simulink model "RV400_Main_Model"  (R2025b)
settings: Solver=VariableStepAuto  StartTime=0.0  StopTime=100  RelTol=1e-3
libraries: fuzblock x1
settings Model: Creator=lenovo  LastModifiedBy=lenovo

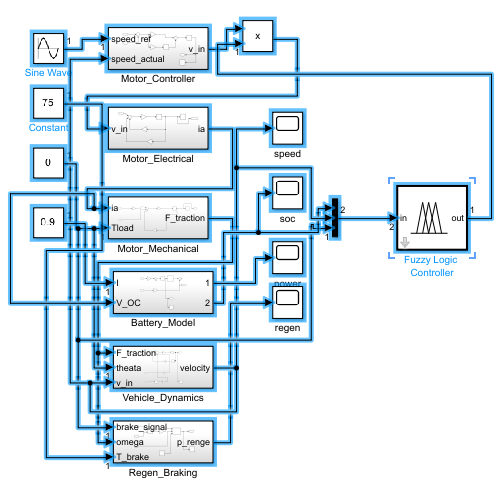
[thumbnail: Simulink's stored preview of the top-level diagram]
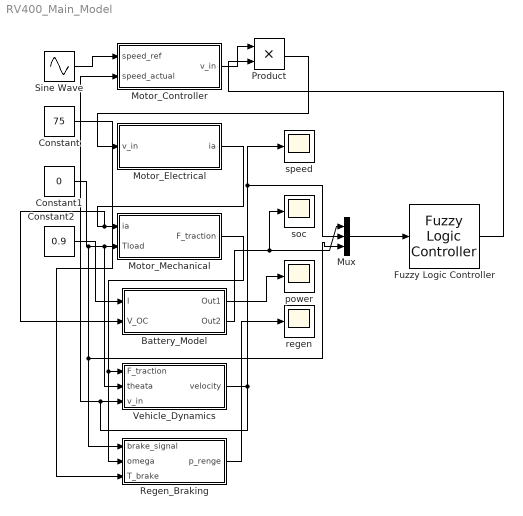
== system RV400_Main_Model ==
  Battery_Model : Subsystem
  Constant : Constant  Value=75
  Constant1 : Constant  Value=0
  Constant2 : Constant  Value=0.9
  Fuzzy Logic Controller : fuzblock/Fuzzy Logic  Controller  FIS=RV400_Fuzzy  OutputSampleNumber=101  DataType=double  UseLookupTable=off  NumBreakpoints=10  FuzzifiedInputs=off  RuleFiringStrengths=off  RuleOutputs=off  AggregatedOutputs=off  SimulateUsing=Interpreted execution  OutOfRangeInputValueMessage=warning  NoRuleFiredMessage=warning  EmptyOutputFuzzySetMessage=warning
  Motor_Controller : Subsystem
  Motor_Electrical : Subsystem
  Motor_Mechanical : Subsystem
  Mux : Mux  Inputs=3
  Product : Product
  Regen_Braking : Subsystem
  Sine Wave : Sin  Amplitude=30  Bias=30  Frequency=0.1  SampleTime=0
  Vehicle_Dynamics : Subsystem
  power : Scope
      settings: ActiveDisplayYMinimum=-0.016951194360907067  ActiveDisplayYMaximum=0.15256074924816365  DataLoggingVariableName=ScopeData2
  regen : Scope
      settings: ActiveDisplayYMinimum=0.9  ActiveDisplayYMaximum=1.1  DataLoggingVariableName=ScopeData3
  soc : Scope
      settings: ActiveDisplayYMinimum=0.89993055555555568  ActiveDisplayYMaximum=0.900624999999999
  speed : Scope
      settings: ActiveDisplayYMinimum=-0.370025922126643  ActiveDisplayYMaximum=3.3302332991397874
  wires:
  Mux/1 -> Fuzzy Logic Controller/1
  Sine Wave/1 -> Motor_Controller/1(speed_ref)
  Motor_Controller/1(v_in) -> Product/1
  Fuzzy Logic Controller/1 -> Product/2
  Product/1 -> Motor_Electrical/1(v_in)
  Motor_Electrical/1(ia) -> Battery_Model/2(V_OC), Motor_Mechanical/1(ia)
  Constant1/1 -> Mux/3, Regen_Braking/1(brake_signal), Vehicle_Dynamics/2(theata), Motor_Mechanical/2(Tload)
  Motor_Mechanical/1(F_traction) -> Regen_Braking/2(omega), Vehicle_Dynamics/1(F_traction)
  Vehicle_Dynamics/1(velocity) -> Mux/2, speed/1, Motor_Controller/2(speed_actual), Vehicle_Dynamics/3(v_in)
  Constant2/1 -> Battery_Model/1(I)
  Battery_Model/1(Out1) -> power/1
  Battery_Model/2(Out2) -> soc/1, Mux/1
  Constant/1 -> Regen_Braking/3(T_brake)
  Regen_Braking/1(p_renge) -> regen/1

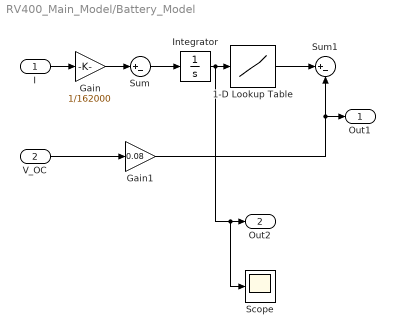
== system RV400_Main_Model/Battery_Model ==
  I : Inport
  V_OC : Inport  Port=2
  1-D Lookup Table : Lookup_n-D  NumberOfTableDimensions=1  BreakpointsForDimension1=[0, 0.2, 0.4, 0.6, 0.8, 0.95, 1.0]  Table=[60.0, 64.8, 68.4, 70.6, 72.9, 75.6, 76.2]  InternalRulePriority=Speed  RndMeth=Simplest
  Gain : Gain  Gain=1/162000
  Gain1 : Gain  Gain=0.08
  Integrator : Integrator  InitialCondition=0.9
  Scope : Scope
      settings: DataLoggingVariableName=ScopeData4
  Sum : Sum  Inputs=|+-
  Sum1 : Sum  Inputs=|+-
  Out1 : Outport
  Out2 : Outport  Port=2
  wires:
  V_OC/1 -> Gain1/1
  Gain1/1 -> Sum1/2, Out1/1
  I/1 -> Gain/1
  Gain/1 -> Sum/1
  1-D Lookup Table/1 -> Sum1/1
  Integrator/1 -> Scope/1, Out2/1, 1-D Lookup Table/1
  Sum/1 -> Integrator/1

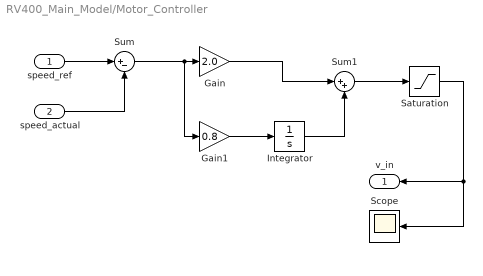
== system RV400_Main_Model/Motor_Controller ==
  speed_ref : Inport
  speed_actual : Inport  Port=2
  Gain : Gain  Gain=2.0
  Gain1 : Gain  Gain=0.8
  Integrator : Integrator
  Saturation : Saturate
  Scope : Scope
      settings: DataLoggingVariableName=ScopeData5
  Sum : Sum  Inputs=|+-
  Sum1 : Sum  Inputs=|++
  v_in : Outport
  wires:
  Integrator/1 -> Sum1/2
  speed_ref/1 -> Sum/1
  Sum1/1 -> Saturation/1
  speed_actual/1 -> Sum/2
  Sum/1 -> Gain1/1, Gain/1
  Gain/1 -> Sum1/1
  Saturation/1 -> v_in/1, Scope/1
  Gain1/1 -> Integrator/1

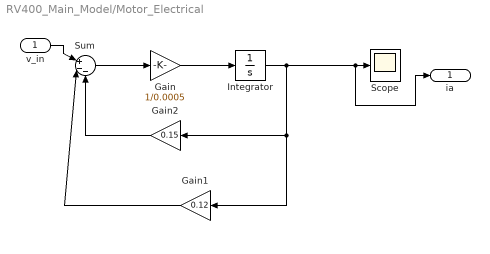
== system RV400_Main_Model/Motor_Electrical ==
  v_in : Inport
  Gain : Gain  Gain=1/0.0005
  Gain1 : Gain  Gain=0.12
  Gain2 : Gain  Gain=0.15
  Integrator : Integrator
  Scope : Scope
      settings: DataLoggingVariableName=ScopeData9
  Sum : Sum  Inputs=|+--
  ia : Outport
  wires:
  Sum/1 -> Gain/1
  Gain/1 -> Integrator/1
  Gain2/1 -> Sum/3
  Gain1/1 -> Sum/2
  Integrator/1 -> ia/1, Scope/1, Gain2/1, Gain1/1
  v_in/1 -> Sum/1

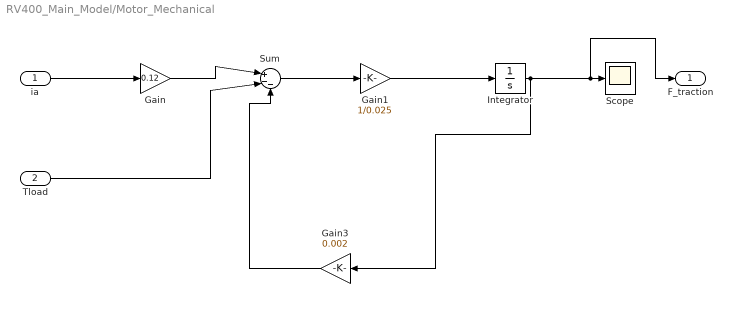
== system RV400_Main_Model/Motor_Mechanical ==
  ia : Inport
  Tload : Inport  Port=2
  Gain : Gain  Gain=0.12
  Gain1 : Gain  Gain=1/0.025
  Gain3 : Gain  Gain=0.002
  Integrator : Integrator
  Scope : Scope
      settings: DataLoggingVariableName=ScopeData8
  Sum : Sum  Inputs=|+--
  F_traction : Outport
  wires:
  Tload/1 -> Sum/2
  Integrator/1 -> Gain3/1, F_traction/1, Scope/1
  Gain3/1 -> Sum/3
  Gain1/1 -> Integrator/1
  Gain/1 -> Sum/1
  ia/1 -> Gain/1
  Sum/1 -> Gain1/1

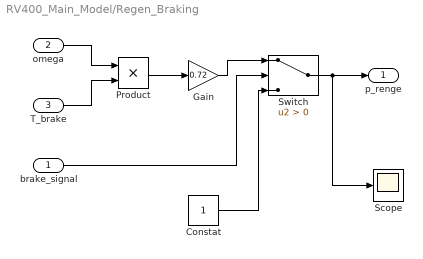
== system RV400_Main_Model/Regen_Braking ==
  brake_signal : Inport
  omega : Inport  Port=2
  T_brake : Inport  Port=3
  Constat : Constant
  Gain : Gain  Gain=0.72
  Product : Product
  Scope : Scope
      settings: DataLoggingVariableName=ScopeData7
  Switch : Switch  Criteria=u2 > Threshold  SaturateOnIntegerOverflow=off  InputSameDT=off
  p_renge : Outport
  wires:
  T_brake/1 -> Product/2
  Switch/1 -> p_renge/1, Scope/1
  Gain/1 -> Switch/1
  Product/1 -> Gain/1
  Constat/1 -> Switch/3
  omega/1 -> Product/1
  brake_signal/1 -> Switch/2

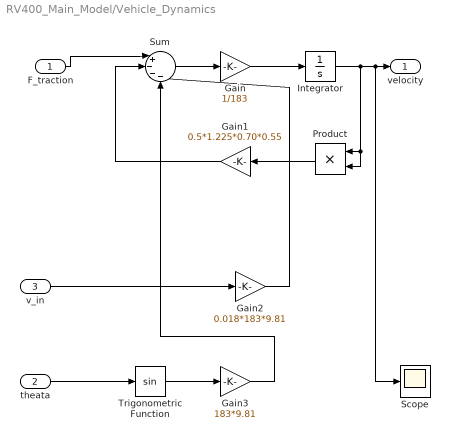
== system RV400_Main_Model/Vehicle_Dynamics ==
  F_traction : Inport
  theata : Inport  Port=2
  v_in : Inport  Port=3
  Gain : Gain  Gain=1/183
  Gain1 : Gain  Gain=0.5*1.225*0.70*0.55
  Gain2 : Gain  Gain=0.018*183*9.81
  Gain3 : Gain  Gain=183*9.81
  Integrator : Integrator
  Product : Product
  Scope : Scope
      settings: DataLoggingVariableName=ScopeData6
  Sum : Sum  Inputs=|+---
  Trigonometric Function : Trigonometry
  velocity : Outport
  wires:
  Gain/1 -> Integrator/1
  Gain2/1 -> Sum/3
  Sum/1 -> Gain/1
  Integrator/1 -> Scope/1, velocity/1, Product/2, Product/1
  Gain3/1 -> Sum/4
  theata/1 -> Trigonometric Function/1
  F_traction/1 -> Sum/1
  Gain1/1 -> Sum/2
  Product/1 -> Gain1/1
  Trigonometric Function/1 -> Gain3/1
  v_in/1 -> Gain2/1
